simulink library "commanapbnd"  (Simulink 5.0)
undefined symbols (not defined in the file or in its folder): den, num
libraries: commutil x4, commanapbnd x3
settings Model: Creator=tdelve  LastModifiedBy=mmclerno

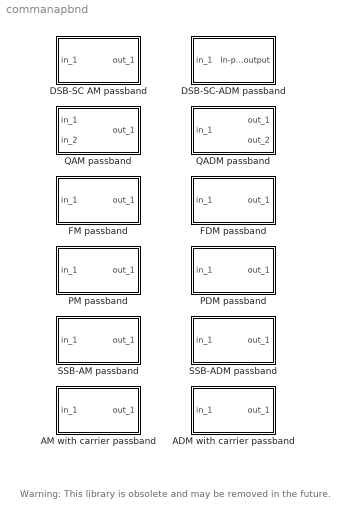
== system commanapbnd ==
  note: Warning:  This library is obsolete and may
      | be removed in the future.
  ADM with carrier passband : Subsystem  mask(Passband ADM with carrier){Offset=1, Fc=100, Ph=0, num=[4.57 9.14 4.57]*.01, den=[1 -1.3108 .4936], ts=0.001}
      mask prompts: Offset "Offset factor:"; Fc "Carrier frequency (Hz):"; Ph "Initial Phase (rad):"; num "Lowpass filter numerator:"; den "Lowpass filter denominator:"; ts "Sample time (sec):"
      mask help: Demodulate an AM with carrier modulated signal.
      mask Help: This block demodulates a DSB-AM with carrier modulated signal. In order to recover the original signal, the offset parameter should be the same as the parameter in the modulation. The demodulation uses a discrete-time lowpass filter that passes the signal message and eliminates the carrier signal.
      mask Display:
      | plot(0,0,100,100,[5+4.5*[0:.3:10] 50 50 50 50+4.5*[0:10]],[85+10*[sin([0:.3:10]*pi/5).*sin([0:.3:10]*pi*2)] 85 99 75 10*sin([0:10]*pi/5)+85]);
      | disp('\nPassband\nADM w TC')
  AM with carrier passband : Subsystem  mask(Passband AM with carrier){Offset=1, Fc=100, Ph=0, ts=0.001}
      mask prompts: Offset "Input signal offset:"; Fc "Carrier frequency (Hz):"; Ph "Initial phase (rad):"; ts "Sample time (sec)"
      mask help: Modulate the input signal using amplitude modulation with transmission carrier method.
      mask Help: This block shifts the amplitude of the input signal before the modulation. AM with carrier is a simple technique but not an energy-efficient one.
      mask Display:
      | plot(0,0,100,100,[4.5*[0:10]+5 50 50 50 50+4.5*[0:.3:10]],[10*sin([0:10]*pi/5)+85 85 99 75 85+10*[sin([0:.3:10]*pi/5).*sin([0:.3:10]*pi*2)]]);
      | disp('\nPassband\nAM w TC')
  DSB-SC AM passband : Subsystem  mask(Passband DSB-SC AM){@1=100, @2=pi/2, @3=0.001}
      mask prompts: @1 "Carrier frequency (Hz):"; @2 "Initial Phase (rad):"; @3 "Sample time (sec):"
      mask help:
      | Modulate the input signal using
      | DSB-SC AM method.
      mask init:
      | Fc=@1;Ph=@2;ts=@3;Fc=Fc*2*pi;
      mask Help: This block modulates the input signal using the double-sideband suppressed-carrier amplitude modulation. In general, the carrier frequency should be much higher than the message signal frequency.
      mask Display:
      | plot(0,0,100,100,[4.5*[0:10]+5 50 50 50 50+4.5*[0:.3:10]],[10*sin([0:10]*pi/5)+85 85 99 75 85+10*[sin([0:.3:10]*pi/5).*sin([0:.3:10]*pi*2)]]);
      | disp('\nPassband\nDSB AM')
  DSB-SC-ADM passband : Subsystem  mask(Passband DSB-SC ADM){@1=100, @2=[4.57 9.14 4.57]*.01, @3=[1 -1.3108 .4936], @4=pi/2, @5=0.001}
      mask prompts: @1 "Carrier frequency (Hz):"; @2 "Lowpass filter numerator:"; @3 "Lowpass filter denominator:"; @4 "Initial phase (rad):"; @5 "Sample time (sec):"
      mask help: Demodulate a DSB-SC AM modulated signal.
      mask init:
      | Fc=@1;num=@2;den=@3;Ph=@4;ts=@5;pi2=pi*2;
      mask Help: This block demodulates a DSB-SC-AM modulated signal using Costas phase-locked loop method. This block uses a discrete-time lowpass filter that passes the signal message and eliminates the carrier signal.
      mask Display:
      | plot(0,0,100,100,[5+4.5*[0:.3:10] 50 50 50 50+4.5*[0:10]],[85+10*[sin([0:.3:10]*pi/5).*sin([0:.3:10]*pi*2)] 85 99 75 10*sin([0:10]*pi/5)+85]);
      | disp('\nPassband\nDSB ADM')
  FDM passband : Subsystem  mask(Passband FDM){Fc=100, Ph=0, HzPerVolt=1, num=[4.57 9.14 4.57]*.01, den=[1 -1.3108 .4936], ts=0.001}
      mask prompts: Fc "Carrier frequency (Hz):"; Ph "Initial phase (rad):"; HzPerVolt "Modulation constant (Hertz per volt):"; num "Lowpass filter numerator:"; den "Lowpass filter denominator:"; ts "Sample time (sec):"
      mask help: Demodulate an FM modulated signal using a phase-locked loop.
      mask init:
      | Ph=Ph+pi/2;
      mask Help: This block recovers a FM modulated signal using a phase-locked loop method. The phase detector used in this block is a multiplier.
      mask Display:
      | plot(0,0,100,100,[5+4.5*[0:.15:10] 50 50 50 50+4.5*[0:10]],[85+10*[sin([0:.15:10]*pi*2+cumsum(sin([0:.15:10]*pi/5))/2)] 85 99 75   10*sin([0:10]*pi/5)+85]);
      | disp('\nPassband\nFDM')
  FM passband : Subsystem  mask(Passband FM){Fc=100, Ph=0, HzPerV=1, ts=0.001, td=Inf}
      mask prompts: Fc "Carrier frequency (Hz):"; Ph "Initial phase (rad):"; HzPerV "Modulation constant (Hertz per volt):"; ts "Sample time (sec):"; td "Symbol interval (sec; Use Inf for analog mod);"
      mask help: Modulate the input signal using FM method.
      mask init:
      | Kc=HzPerV;pi2=2*pi;if isinf(td),td=realmax;end;
      mask Help: This block modulates the input signal using frequency modulation method. The frequency of the output of the carrier signal depends on the amplitude of the input signal.
      mask Display:
      | plot(0,0,100,100,[4.5*[0:10]+5 50 50 50 50+4.5*[0:.15:10]],[10*sin([0:10]*pi/5)+85 85 99 75 85+10*[sin([0:.15:10]*pi*2+cumsum(sin([0:.15:10]*pi/5))/2)]]);
      | disp('\nPassband\nFM')
  PDM passband : Subsystem  mask(Passband PDM){Fc=100, Ph=0, Kc=1, num=[4.57 9.14 4.57]*.01, den=[1 -1.3108 .4936], HzPerVolt=1, ts=0.001}
      mask prompts: Fc "Carrier frequency (Hz):"; Ph "Initial phase (rad):"; Kc "Modulation constant (Radians per volt):"; num "Lowpass filter numerator:"; den "Lowpass filter denominator:"; HzPerVolt "VCO Gain (Hertz per volt):"; ts "Sample time (sec):"
      mask help: Demodulate a PM modulated signal using a phase locked loop.
      mask init:
      | Ph=Ph+pi/2;
      | Kv=2*pi*HzPerVolt;
      mask Help: This block recovers a PM modulated signal. This block uses a multiplier phase detector in PLL. This block uses a discrete-time lowpass filter which passes the signal message and eliminates the carrier signal.
      mask Display:
      | plot(0,0,100,100,[5+4.5*[0:.15:10] 50 50 50 50+4.5*[0:10]],[85+10*[sin([0:.15:10]*pi*2+cumsum(sin([0:.15:10]*pi/5))/2)] 85 99 75   10*sin([0:10]*pi/5)+85]);
      | disp('\nPassband\nPDM')
  PM passband : Subsystem  mask(Passband PM){Fc=100, Ph=0, Kc=1, td=Inf}
      mask prompts: Fc "Carrier frequency (Hz):"; Ph "Initial phase (rad):"; Kc "Modulation constant (Radians per volt):"; td "Symbol interval (sec, Use inf for analog case):"
      mask help: Modulate the input signal using PM method.
      mask init:
      | Fc=Fc*2*pi;if isinf(td),td=realmax;end;
      mask Help: The PM block causes the change of the carrier signal depending on the input signal voltage.
      mask Display:
      | plot(0,0,100,100,[4.5*[0:10]+5 50 50 50 50+4.5*[0:.15:10]],[10*sin([0:10]*pi/5)+85 85 99 75 85+10*[sin([0:.15:10]*pi*2+cumsum(sin([0:.15:10]*pi/5))/2)]]);
      | disp('\nPassband\nPM')
  QADM passband : Subsystem  mask(Passband DSB-SC QADM){Fc=100, num=[4.57 9.14 4.57]*.01, den=[1 -1.3108 .4936], Ph=0, ts=0.001}
      mask prompts: Fc "Carrier frequency (Hz):"; num "Lowpass filter numerator:"; den "Lowpass filter denominator:"; Ph "Initial phase (rad):"; ts "Sample time (sec):"
      mask help: Demodulate a DSB-SC QAM modulated signal into in-phase and quadrature components.
      mask init:
      | Fc=Fc*2*pi;
      mask Help: This block demodulates the QM-DSB-SC-AM modulated signal. The first output port outputs the in-phase component and the second port outputs the quadrature component. The demodulation uses a discrete-time lowpass filter that passes the signal message and eliminates the carrier signal.
      mask Display:
      | plot(0,0,100,100,[5+4.5*[0:.3:10] 50 50 50 50+4.5*[0:10]],[85+10*[sin([0:.3:10]*pi/5).*sin([0:.3:10]*pi*2)] 85 99 75 10*sin([0:10]*pi/5)+85]);
      | disp('\nPassband\nQADM')
  QAM passband : Subsystem  mask(Passband DSB-SC QAM){Fc=100, Ph=0, ts=0.001}
      mask prompts: Fc "Carrier frequency (Hz):"; Ph "Initial phase (rad):"; ts "Sample time (sec):"
      mask help: Modulate the in-phase signal from first input port and quadrature signal from the second port using QAM.
      mask init:
      | Fc=Fc*2*pi;
      mask Help: This block modulates the in-phase component input from the first port and the quadrature component input from the second port by using two orthogonal sinusoidal carriers.
      mask Display:
      | plot(0,0,100,100,[4.5*[0:10]+5 50 50 50 50+4.5*[0:.3:10]],[10*sin([0:10]*pi/5)+85 85 99 75 85+10*[sin([0:.3:10]*pi/5).*sin([0:.3:10]*pi*2)]]);
      | disp('\nPassband\nQAM')
  SSB-ADM passband : Subsystem  mask(Passband SSB ADM){@1=100, @2=[4.57 9.14 4.57]*.01, @3=[1 -1.3108 .4936], @4=0, @5=0.001}
      mask prompts: @1 "Carrier frequency (Hz):"; @2 "Lowpass filter numerator:"; @3 "Lowpass filter denominator:"; @4 "Initial phase (rad):"; @5 "Sample time (sec):"
      mask help: Demodulate a SSB-AM modulated signal.
      mask init:
      | Fc=@1;num=@2;den=@3;Ph=@4;ts=@5;Fc=Fc*2*pi;Pg=Ph+pi/2;
      mask Help: This block demodulates the SSB-SC-AM modulated signal. The demodulation uses a discrete-time lowpass filter that passes the signal message and eliminates the carrier signal. You can specify the modulation to be a USB or LSB modulation.
      mask Display:
      | plot(0,0,100,100,[5+4.5*[0:.3:10] 50 50 50 50+4.5*[0:10]],[85+10*[sin([0:.3:10]*pi/5).*sin([0:.3:10]*pi*2)] 85 99 75 10*sin([0:10]*pi/5)+85]);
      | disp('\nPassband\nSSB ADM')
  SSB-AM passband : Subsystem  mask(Passband SSB-AM){Fc=100, Ph=0, ban=1/.01/10, dly=0.01, ts=0.001, sd='upper'}
      mask prompts: Fc "Carrier frequency (Hz):"; Ph "Initial Phase (rad):"; ban "Bandwidth of the input signal (Hz):"; dly "Time delay for Hilbert transform filter (sec):"; ts "Sample time (sec):"; sd ""upper" sideband or "lower" sideband:"
      mask help: Modulate the input signal using single-sideband amplitude modulation method with Hilbert transform filter.
      mask init:
      | if ban>1/ts, ban=1/ts-ts;end;[num,den]=hilbiir(ts,dly,ban);pi2=2*pi;pih=pi/2;k=-1;if sd(1)=='l',k=1;end;
      mask Help: This block modulates the input signal using the SSB-AM method. The block uses Hilbert transfer filter. Hilbert transform filter is a non-causal filter. A positive time delay is requested in the implementation. You can specify the modulation to be an USB or LSB modulation.
      mask Display:
      | plot(0,0,100,100,[4.5*[0:10]+5 50 50 50 50+4.5*[0:.3:10]],[10*sin([0:10]*pi/5)+85 85 99 75 85+10*[sin([0:.3:10]*pi/5).*sin([0:.3:10]*pi*2)]]);
      | disp('\nPassband\nSSB AM')

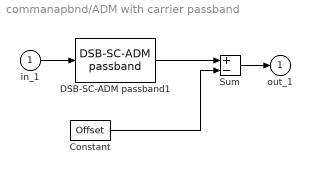
== system commanapbnd/ADM with carrier passband ==
  in_1 : Inport
  Constant : Constant  Value=Offset
  DSB-SC-ADM passband1 : commanapbnd/DSB-SC-ADM passband  MaskParam1=Fc  MaskParam2=num  MaskParam3=den  MaskParam4=Ph  MaskParam5=ts
  Sum : Sum  Inputs=+-  SaturateOnIntegerOverflow=on  InputSameDT=on
  out_1 : Outport  InitialOutput=0
  wires:
  Constant/1 -> Sum/2
  Sum/1 -> out_1/1
  DSB-SC-ADM passband1/1 -> Sum/1
  in_1/1 -> DSB-SC-ADM passband1/1

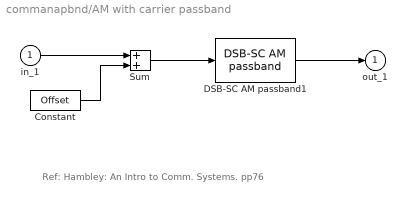
== system commanapbnd/AM with carrier passband ==
  note: Ref: Hambley: An Intro to Comm. Systems. pp76
  in_1 : Inport
  Constant : Constant  Value=Offset
  DSB-SC AM passband1 : commanapbnd/DSB-SC AM passband  MaskParam1=Fc  MaskParam2=Ph  MaskParam3=ts
  Sum : Sum  SaturateOnIntegerOverflow=on  InputSameDT=on
  out_1 : Outport  InitialOutput=0
  wires:
  Constant/1 -> Sum/2
  DSB-SC AM passband1/1 -> out_1/1
  Sum/1 -> DSB-SC AM passband1/1
  in_1/1 -> Sum/1

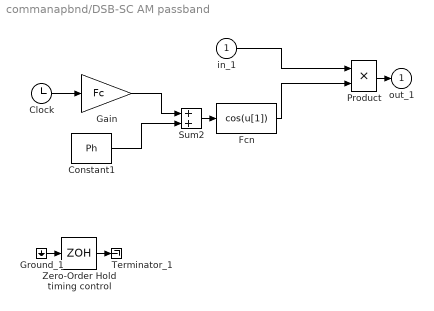
== system commanapbnd/DSB-SC AM passband ==
  in_1 : Inport
  Clock : Clock
      settings: Decimation=10
  Constant1 : Constant  Value=Ph
  Fcn : Fcn  Expr=cos(u[1])
  Gain : Gain  Gain=Fc  SaturateOnIntegerOverflow=on
  Ground_1 : Ground
  Product : Product  SaturateOnIntegerOverflow=on  InputSameDT=on
  Sum2 : Sum  SaturateOnIntegerOverflow=on  InputSameDT=on
  Terminator_1 : Terminator
  Zero-Order Hold timing control : ZeroOrderHold  SampleTime=ts
  out_1 : Outport  InitialOutput=0
  wires:
  Zero-Order Hold timing control/1 -> Terminator_1/1
  Ground_1/1 -> Zero-Order Hold timing control/1
  Fcn/1 -> Product/2
  Product/1 -> out_1/1
  in_1/1 -> Product/1
  Clock/1 -> Gain/1
  Gain/1 -> Sum2/1
  Constant1/1 -> Sum2/2
  Sum2/1 -> Fcn/1

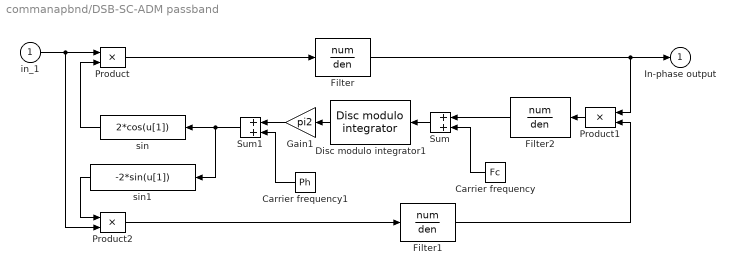
== system commanapbnd/DSB-SC-ADM passband ==
  in_1 : Inport
  Carrier frequency : Constant  Orientation=left  Value=Fc
  Carrier frequency1 : Constant  Orientation=left  Value=Ph
  Disc modulo integrator1 : commutil/Disc modulo integrator  Orientation=left  modu=1  init=0  ts=ts
  Filter : DiscreteFilter  Numerator=num  Denominator=den  SampleTime=ts
  Filter1 : DiscreteFilter  Numerator=num  Denominator=den  SampleTime=ts
  Filter2 : DiscreteFilter  Orientation=left  Numerator=num  Denominator=den  SampleTime=ts
  Gain1 : Gain  Orientation=left  Gain=pi2  SaturateOnIntegerOverflow=on
  Product : Product  SaturateOnIntegerOverflow=on  InputSameDT=on
  Product1 : Product  Orientation=left  SaturateOnIntegerOverflow=on  InputSameDT=on
  Product2 : Product  SaturateOnIntegerOverflow=on  InputSameDT=on
  Sum : Sum  Orientation=left  SaturateOnIntegerOverflow=on  InputSameDT=on
  Sum1 : Sum  Orientation=left  SaturateOnIntegerOverflow=on  InputSameDT=on
  sin : Fcn  Orientation=left  Expr=2*cos(u[1])
  sin1 : Fcn  Orientation=left  Expr=-2*sin(u[1])
  In-phase output : Outport  InitialOutput=0
  wires:
  Sum1/1 -> sin/1, sin1/1
  Filter2/1 -> Sum/1
  Product/1 -> Filter/1
  sin/1 -> Product/2
  Carrier frequency/1 -> Sum/2
  Sum/1 -> Disc modulo integrator1/1
  Product1/1 -> Filter2/1
  sin1/1 -> Product2/1
  in_1/1 -> Product/1, Product2/2
  Product2/1 -> Filter1/1
  Filter1/1 -> Product1/2
  Disc modulo integrator1/1 -> Gain1/1
  Gain1/1 -> Sum1/1
  Carrier frequency1/1 -> Sum1/2
  Filter/1 -> In-phase output/1, Product1/1

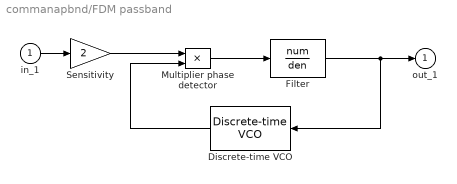
== system commanapbnd/FDM passband ==
  in_1 : Inport
  Discrete-time VCO : commutil/Discrete-time VCO  Orientation=left  Ac=1  Fc=Fc  Kc=HzPerVolt  Ph=Ph  ts=ts
  Filter : DiscreteFilter  Numerator=num  Denominator=den  SampleTime=ts
  Multiplier phase detector : Product  SaturateOnIntegerOverflow=on  InputSameDT=on
  Sensitivity : Gain  Gain=2  SaturateOnIntegerOverflow=on
  out_1 : Outport  InitialOutput=0
  wires:
  Discrete-time VCO/1 -> Multiplier phase detector/2
  Multiplier phase detector/1 -> Filter/1
  Filter/1 -> out_1/1, Discrete-time VCO/1
  in_1/1 -> Sensitivity/1
  Sensitivity/1 -> Multiplier phase detector/1

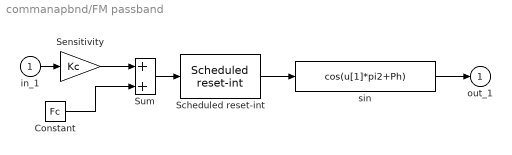
== system commanapbnd/FM passband ==
  in_1 : Inport
  Constant : Constant  Value=Fc
  Scheduled reset-int : commutil/Scheduled reset-int  td=td  ts=ts  limit=Inf/2
  Sensitivity : Gain  Gain=Kc  SaturateOnIntegerOverflow=on
  Sum : Sum  SaturateOnIntegerOverflow=on  InputSameDT=on
  sin : Fcn  Expr=cos(u[1]*pi2+Ph)
  out_1 : Outport  InitialOutput=0
  wires:
  sin/1 -> out_1/1
  Scheduled reset-int/1 -> sin/1
  Sum/1 -> Scheduled reset-int/1
  Constant/1 -> Sum/2
  in_1/1 -> Sensitivity/1
  Sensitivity/1 -> Sum/1

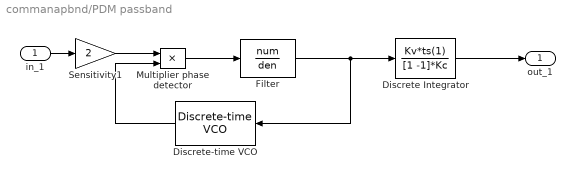
== system commanapbnd/PDM passband ==
  in_1 : Inport
  Discrete Integrator : DiscreteFilter  Numerator=Kv*ts(1)  Denominator=[1 -1]*Kc  SampleTime=ts
  Discrete-time VCO : commutil/Discrete-time VCO  Orientation=left  Ac=1  Fc=Fc  Kc=HzPerVolt  Ph=Ph  ts=ts
  Filter : DiscreteFilter  Numerator=num  Denominator=den  SampleTime=ts
  Multiplier phase detector : Product  SaturateOnIntegerOverflow=on  InputSameDT=on
  Sensitivity1 : Gain  Gain=2  SaturateOnIntegerOverflow=on
  out_1 : Outport  InitialOutput=0
  wires:
  Discrete-time VCO/1 -> Multiplier phase detector/2
  Filter/1 -> Discrete-time VCO/1, Discrete Integrator/1
  Discrete Integrator/1 -> out_1/1
  Multiplier phase detector/1 -> Filter/1
  in_1/1 -> Sensitivity1/1
  Sensitivity1/1 -> Multiplier phase detector/1

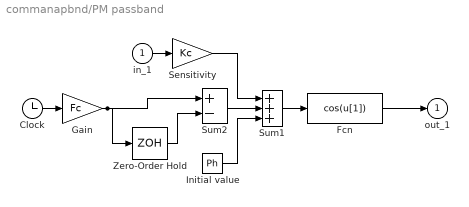
== system commanapbnd/PM passband ==
  in_1 : Inport
  Clock : Clock
      settings: Decimation=10
  Fcn : Fcn  Expr=cos(u[1])
  Gain : Gain  Gain=Fc  SaturateOnIntegerOverflow=on
  Initial value : Constant  Value=Ph
  Sensitivity : Gain  Gain=Kc  SaturateOnIntegerOverflow=on
  Sum1 : Sum  Inputs=+++  SaturateOnIntegerOverflow=on  InputSameDT=on
  Sum2 : Sum  Inputs=+-  SaturateOnIntegerOverflow=on  InputSameDT=on
  Zero-Order Hold : ZeroOrderHold  SampleTime=td
  out_1 : Outport  InitialOutput=0
  wires:
  Fcn/1 -> out_1/1
  Initial value/1 -> Sum1/3
  Sum1/1 -> Fcn/1
  Clock/1 -> Gain/1
  Sum2/1 -> Sum1/2
  Zero-Order Hold/1 -> Sum2/2
  Gain/1 -> Sum2/1, Zero-Order Hold/1
  in_1/1 -> Sensitivity/1
  Sensitivity/1 -> Sum1/1

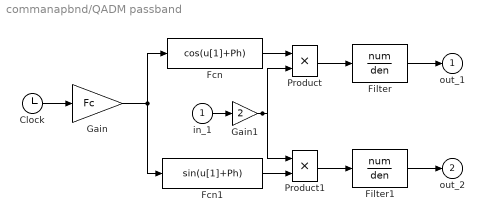
== system commanapbnd/QADM passband ==
  in_1 : Inport
  Clock : Clock
      settings: Decimation=10
  Fcn : Fcn  Expr=cos(u[1]+Ph)
  Fcn1 : Fcn  Expr=sin(u[1]+Ph)
  Filter : DiscreteFilter  Numerator=num  Denominator=den  SampleTime=ts
  Filter1 : DiscreteFilter  Numerator=num  Denominator=den  SampleTime=ts
  Gain : Gain  Gain=Fc  SaturateOnIntegerOverflow=on
  Gain1 : Gain  Gain=2  SaturateOnIntegerOverflow=on
  Product : Product  SaturateOnIntegerOverflow=on  InputSameDT=on
  Product1 : Product  SaturateOnIntegerOverflow=on  InputSameDT=on
  out_1 : Outport  InitialOutput=0
  out_2 : Outport  Port=2  InitialOutput=0
  wires:
  Clock/1 -> Gain/1
  Filter1/1 -> out_2/1
  Product1/1 -> Filter1/1
  Filter/1 -> out_1/1
  Product/1 -> Filter/1
  Fcn1/1 -> Product1/2
  Fcn/1 -> Product/1
  Gain/1 -> Fcn/1, Fcn1/1
  in_1/1 -> Gain1/1
  Gain1/1 -> Product/2, Product1/1

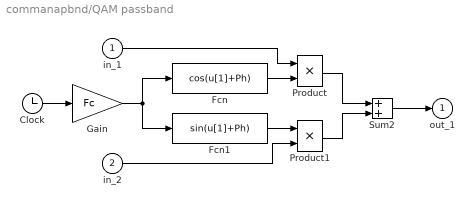
== system commanapbnd/QAM passband ==
  in_1 : Inport
  in_2 : Inport  Port=2
  Clock : Clock
      settings: Decimation=10
  Fcn : Fcn  Expr=cos(u[1]+Ph)
  Fcn1 : Fcn  Expr=sin(u[1]+Ph)
  Gain : Gain  Gain=Fc  SaturateOnIntegerOverflow=on
  Product : Product  SaturateOnIntegerOverflow=on  InputSameDT=on
  Product1 : Product  SaturateOnIntegerOverflow=on  InputSameDT=on
  Sum2 : Sum  SaturateOnIntegerOverflow=on  InputSameDT=on
  out_1 : Outport  InitialOutput=0
  wires:
  Gain/1 -> Fcn/1, Fcn1/1
  Clock/1 -> Gain/1
  Product1/1 -> Sum2/2
  Product/1 -> Sum2/1
  in_2/1 -> Product1/2
  Fcn1/1 -> Product1/1
  in_1/1 -> Product/1
  Fcn/1 -> Product/2
  Sum2/1 -> out_1/1

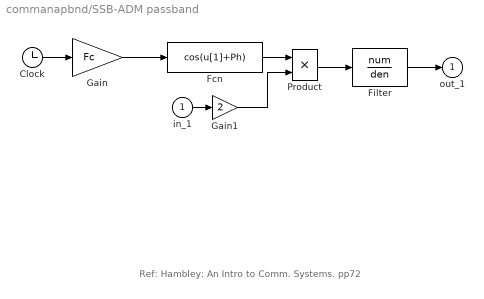
== system commanapbnd/SSB-ADM passband ==
  note: Ref: Hambley: An Intro to Comm. Systems. pp72
  in_1 : Inport
  Clock : Clock
      settings: Decimation=10
  Fcn : Fcn  Expr=cos(u[1]+Ph)
  Filter : DiscreteFilter  Numerator=num  Denominator=den  SampleTime=ts
  Gain : Gain  Gain=Fc  SaturateOnIntegerOverflow=on
  Gain1 : Gain  Gain=2  SaturateOnIntegerOverflow=on
  Product : Product  SaturateOnIntegerOverflow=on  InputSameDT=on
  out_1 : Outport  InitialOutput=0
  wires:
  Clock/1 -> Gain/1
  Filter/1 -> out_1/1
  Product/1 -> Filter/1
  Fcn/1 -> Product/1
  in_1/1 -> Gain1/1
  Gain1/1 -> Product/2
  Gain/1 -> Fcn/1

== system commanapbnd/SSB-AM passband ==
  in_1 : Inport
  Filter : DiscreteFilter  Numerator=num  Denominator=den  SampleTime=ts
  Gain : Gain  Gain=k  SaturateOnIntegerOverflow=on
  QAM passband : commanapbnd/QAM passband  Fc=Fc  Ph=Ph  ts=ts
  out_1 : Outport  InitialOutput=0
  wires:
  QAM passband/1 -> out_1/1
  in_1/1 -> QAM passband/1, Filter/1
  Filter/1 -> Gain/1
  Gain/1 -> QAM passband/2
